simulink model "a2lathos"  (R2020a)
settings: Solver=VariableStepAuto  StartTime=0.0  StopTime=1  RelTol=1e-3
settings Model: Creator=bill2  LastModifiedBy=bill2
settings DataIOCC: Refine=10

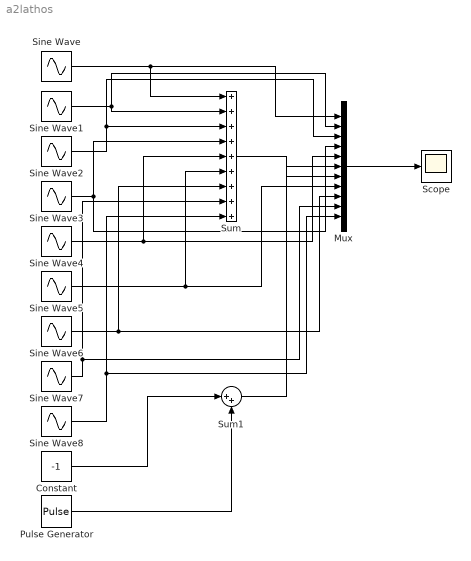
== system a2lathos ==
  Constant : Constant  Value=-1
  Mux : Mux  Inputs=11
  Pulse Generator : DiscretePulseGenerator  PulseType=Time based  Amplitude=2  Period=10  PulseWidth=5  PhaseDelay=0.001  VectorParams1D=off
  Scope : Scope
  Sine Wave : Sin  Amplitude=4/pi  Frequency=2*pi  SampleTime=0
  Sine Wave1 : Sin  Amplitude=4/(3*pi)  Frequency=6*pi  SampleTime=0
  Sine Wave2 : Sin  Amplitude=4/(5*pi)  Frequency=10*pi  SampleTime=0
  Sine Wave3 : Sin  Amplitude=4/(7*pi)  Frequency=14*pi  SampleTime=0
  Sine Wave4 : Sin  Amplitude=4/(9*pi)  Frequency=18*pi  SampleTime=0
  Sine Wave5 : Sin  Amplitude=4/(11*pi)  Frequency=22*pi  SampleTime=0
  Sine Wave6 : Sin  Amplitude=4/(13*pi)  Frequency=26*pi  SampleTime=0
  Sine Wave7 : Sin  Amplitude=4/(15*pi)  Frequency=30*pi  SampleTime=0
  Sine Wave8 : Sin  Amplitude=4/(17*pi)  Frequency=33*pi  SampleTime=0
  Sum : Sum  Inputs=9
  Sum1 : Sum  Inputs=|++
  wires:
  Sine Wave/1 -> Mux/1, Sum/1
  Sine Wave1/1 -> Mux/2, Sum/2
  Sine Wave2/1 -> Mux/3, Sum/3
  Sine Wave3/1 -> Mux/4, Sum/4
  Sine Wave4/1 -> Mux/5, Sum/5
  Sum/1 -> Mux/7
  Constant/1 -> Sum1/1
  Sum1/1 -> Mux/6
  Sine Wave5/1 -> Mux/8, Sum/6
  Sine Wave6/1 -> Sum/7, Mux/9
  Sine Wave7/1 -> Mux/10, Sum/8
  Sine Wave8/1 -> Mux/11, Sum/9
  Pulse Generator/1 -> Sum1/2
  Mux/1 -> Scope/1
